simulink model "NonLinear"  (R2016a)
settings: Solver=VariableStepAuto  StartTime=0.0  StopTime=10.0  RelTol=1e-3
settings Model: Creator=asus  LastModifiedBy=asus

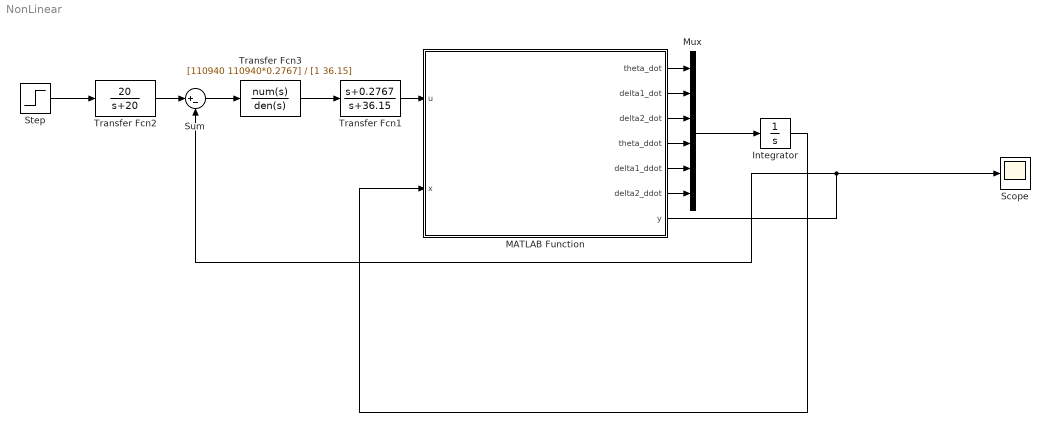
== system NonLinear ==
  Integrator : Integrator  InitialCondition=zeros(6,1)
  MATLAB Function : MATLAB Function  TreatAsAtomicUnit=on
  Mux : Mux  Inputs=6
  Scope : Scope
  Step : Step  SampleTime=0
  Sum : Sum  Inputs=|+-
  Transfer Fcn1 : TransferFcn  Numerator=[1 0.2767]  Denominator=[1 36.15]
  Transfer Fcn2 : TransferFcn  Numerator=[20]  Denominator=[1 20]
  Transfer Fcn3 : TransferFcn  Numerator=[110940 110940*0.2767]  Denominator=[1 36.15]
  wires:
  MATLAB Function/1(theta_dot) -> Mux/1
  MATLAB Function/2(delta1_dot) -> Mux/2
  MATLAB Function/3(delta2_dot) -> Mux/3
  MATLAB Function/4(theta_ddot) -> Mux/4
  MATLAB Function/5(delta1_ddot) -> Mux/5
  MATLAB Function/6(delta2_ddot) -> Mux/6
  Integrator/1 -> MATLAB Function/2(x)
  MATLAB Function/7(y) -> Scope/1, Sum/2
  Mux/1 -> Integrator/1
  Transfer Fcn2/1 -> Sum/1
  Step/1 -> Transfer Fcn2/1
  Transfer Fcn3/1 -> Transfer Fcn1/1
  Sum/1 -> Transfer Fcn3/1
  Transfer Fcn1/1 -> MATLAB Function/1(u)

== matlab function NonLinear/MATLAB Function ==
  data: u input; theta_dot output; x input; delta1_dot output; delta2_dot output; theta_ddot output; delta1_ddot output; delta2_ddot output; y output
function [theta_dot, delta1_dot, delta2_dot, theta_ddot, delta1_ddot, delta2_ddot,y] = fcn(u,x)
%#codegen
%Parameters from Table 2.1
l     = 1.2     ; % Length of link
Gamma = 1.2     ; % Gamma = pA
b     = 0.59    ; % b = F1;
EI    = 1.94    ; % = E*I;
w1    = 3       ; % Frequency of delta1
w2    = 19      ; % Frequency of delta2
c1    = 0.4     ; % Constant in phi1 formula that normalizes the eigenfunction
c2    = 4       ; % Constant in phi2 formula that normalizes the eigenfunction
a     = 0.6     ; % The ratio for stabilizing the system
f1    = 2.5     ; % First element of F2 matrix
f2    = 9     ; % Second element of F2 matrix
k1    = 17.4561 ; % First element of K matrix
k2    = 685.5706; % Second element of K matrix
Ccoul = 4.8     ;

%Defining M matrix from appendix B
M = [ 0.9929+0.12*(x(2)-x(3))^2   1.0703  -0.0282;
      1.0703                      1.6235  -0.4241;
     -0.0282                     -0.4241   2.5920];
 
Minv = inv(M);

%Defining F2 matrix
F2 = [f1 0;
      0  f2];
%Defining K matrix  
K = [k1  0;
      0  k2];
  
%Definig h1
h1 = 0.24*x(4)*((x(2)-x(3))*x(5)-(x(2)-x(3))*x(6));
%Definig h2
h2 = [-0.12*x(4)^2*(x(2)-x(3));
      -0.12*x(4)^2*(x(3)-x(2))];
%Definig fc
fc = Ccoul*(2/(1+exp(-10*x(4)))-1);

%Dedining D matrix
D = [h1+b*x(4)+fc;
     h2(1)+k1*x(2)+f1*x(5);
     h2(2)+k2*x(3)+f2*x(6)];

A = -Minv*D; 
B = Minv*[u;0;0];

 beta1 = sqrt(w1*(sqrt(Gamma*l^4/EI)));
 beta2 = sqrt(w2*(sqrt(Gamma*l^4/EI)));
 phi1  = c1*((sin(beta1*l)-sinh(beta1*l)) - (sin(beta1*l)+sinh(beta1*l))*(cos(beta1*l)-cosh(beta1*l))/(cos(beta1*l)+cosh(beta1*l)));
 phi2  = c2*((sin(beta2*l)-sinh(beta2*l)) - (sin(beta2*l)+sinh(beta2*l))*(cos(beta2*l)-cosh(beta2*l))/(cos(beta2*l)+cosh(beta2*l)));


theta_ddot  = A(1) +B(1);
delta1_ddot = A(2) +B(2);
delta2_ddot = A(3) +B(3);
theta_dot  = x(4);
delta1_dot = x(5);
delta2_dot = x(6);
y = x(1) + a*phi1/l*x(2) + a*phi2/l*x(3);
